simulink model "time_delay"  (R2015a)
settings: Solver=ode45  StartTime=0.0  StopTime=3  RelTol=1e-3
libraries: cstblocks x3
settings Model: Creator=Kripa95  LastModifiedBy=dj

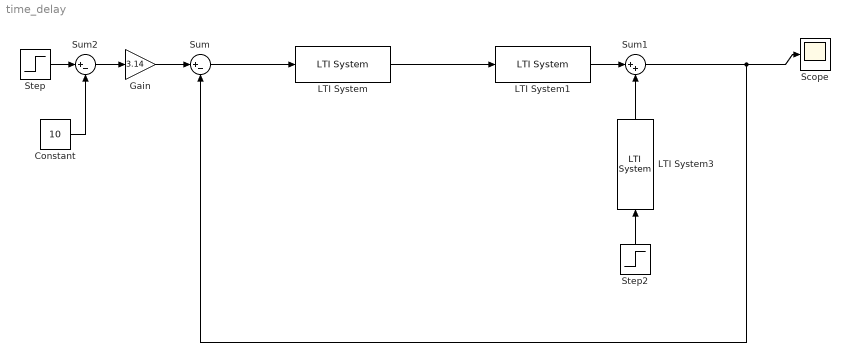
== system time_delay ==
  Constant : Constant  Value=10
  Gain : Gain  Gain=3.14
  LTI System : cstblocks/LTI System  sys=C  IC=[]
  LTI System1 : cstblocks/LTI System  sys=G  IC=[]
  LTI System3 : cstblocks/LTI System  sys=t_d  IC=[]
  Scope : Scope
      settings: YMin=-6  YMax=1
  Step : Step  Time=0  After=12  SampleTime=0
  Step2 : Step  Time=2  SampleTime=0
  Sum : Sum  Inputs=|+-
  Sum1 : Sum  Inputs=|++
  Sum2 : Sum  Inputs=|+-
  wires:
  LTI System1/1 -> Sum1/1
  Sum1/1 -> Sum/2, Scope/1
  LTI System3/1 -> Sum1/2
  Step2/1 -> LTI System3/1
  Sum/1 -> LTI System/1
  LTI System/1 -> LTI System1/1
  Gain/1 -> Sum/1
  Step/1 -> Sum2/1
  Sum2/1 -> Gain/1
  Constant/1 -> Sum2/2
